simulink model "QUESTION3_4"  (R2021a)
settings: Solver=VariableStepAuto  StartTime=0.0  StopTime=10.0  RelTol=1e-3
settings Model: Creator=user  LastModifiedBy=user

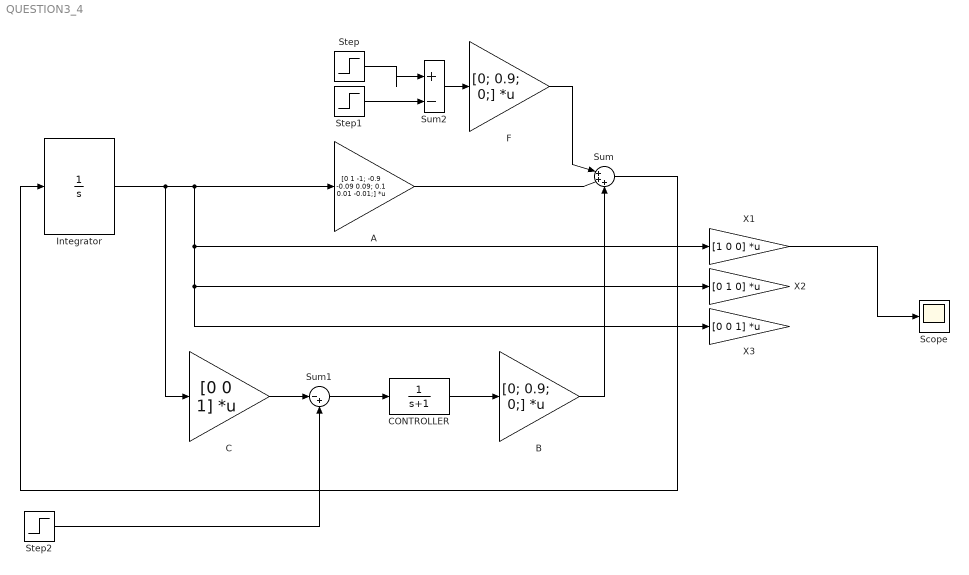
== system QUESTION3_4 ==
  A : Gain  Gain=[0 1 -1; -0.9 -0.09 0.09; 0.1 0.01 -0.01;]  Multiplication=Matrix(K*u)
  B : Gain  Gain=[0; 0.9; 0;]  Multiplication=Matrix(K*u)
  C : Gain  Gain=[0 0 1]  Multiplication=Matrix(K*u)
  CONTROLLER : TransferFcn  Denominator=[1 1]
  F : Gain  Gain=[0; 0.9; 0;]  Multiplication=Matrix(K*u)
  Integrator : Integrator
  Scope : Scope
  Step : Step  Time=20  SampleTime=0
  Step1 : Step  Time=22  SampleTime=0
  Step2 : Step  Time=0  SampleTime=0
  Sum : Sum  Inputs=|+++
  Sum1 : Sum  Inputs=|-+
  Sum2 : Sum  Inputs=|+-
  X1 : Gain  Gain=[1 0 0]  Multiplication=Matrix(K*u)
  X2 : Gain  Gain=[0 1 0]  Multiplication=Matrix(K*u)
  X3 : Gain  Gain=[0 0 1]  Multiplication=Matrix(K*u)
  wires:
  Integrator/1 -> X3/1, X2/1, X1/1, A/1, C/1
  CONTROLLER/1 -> B/1
  B/1 -> Sum/3
  A/1 -> Sum/2
  Sum/1 -> Integrator/1
  C/1 -> Sum1/1
  Sum1/1 -> CONTROLLER/1
  Step1/1 -> Sum2/2
  Step/1 -> Sum2/1
  Sum2/1 -> F/1
  F/1 -> Sum/1
  Step2/1 -> Sum1/2
  X1/1 -> Scope/1
